simulink model "cm10"  (R2015b)
settings: Solver=VariableStepAuto  StartTime=0.0  StopTime=100  RelTol=1e-3
settings Model: Creator=Zephyr  LastModifiedBy=Zephyr

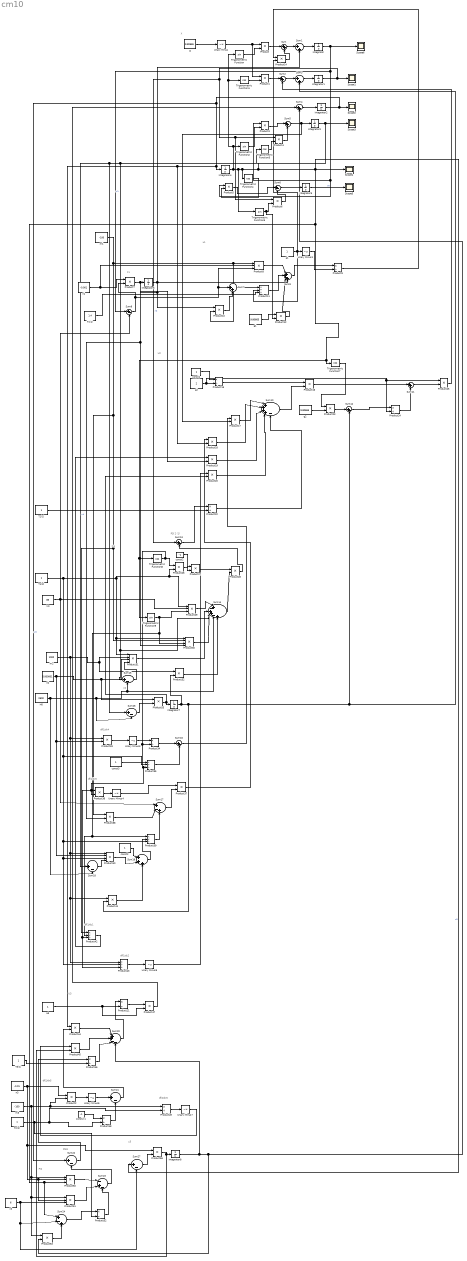
== system cm10 ==
  note: u1
  note: z3
  note: z2
  note: z1
  note: FI2
  note: PSI3
  note: dfi2/dx5
  note: dfi2/dx5
  note: U3
  note: dfi1/dz2
  note: dfi1/dz1
  note: dfi1/dx5
  note: dfi1/dx4
  note: FI1
  note: PSI 2 (1)
  note: U2
  note: X
  H0 : Constant  Value=2600
  Integrator{,1..8} (9 alike) : Integrator
  Product{,1..7,10,12,14,16..20,23,25..28,32..33,36..38,41,44..45,47,53,55..56} (33 alike) : Product
  Product11 : Product  Inputs=*//
  Product{9,15,21..22,24,34,46,48..49,52} (10 alike) : Product  Inputs=*/
  Product{8,29,50..51} (4 alike) : Product  Inputs=3
  Product30 : Product  Inputs=4
  Product31 : Product  Inputs=4
  Product35 : Product  Inputs=*//
  Product39 : Product  Inputs=**/
  Product40 : Product  Inputs=4
  Product42 : Product  Inputs=**/
  Product43 : Product  Inputs=*//
  Scope{1..6} (6 alike) : Scope
  Sum{,1..5,7,11} (8 alike) : Sum  Inputs=|++
  Sum10 : Sum  Inputs=|++++-
  Sum{6,8,12..13,15..16,18,21..22,26..27} (11 alike) : Sum  Inputs=|+-
  Sum14 : Sum  Inputs=|+-++-+
  Sum17 : Sum  Inputs=|+-+
  Sum19 : Sum  Inputs=|+++
  Sum20 : Sum  Inputs=|++--
  Sum23 : Sum  Inputs=|-+-
  Sum24 : Sum  Inputs=|+-+
  Sum9 : Sum  Inputs=|++-+
  T1(1) : Constant  Value=1.4
  T1(2) : Constant
  T2(1) : Constant
  T2(2) : Constant
  T3(1) : Constant
  Trigonometric Function{,2,5,9} (4 alike) : Trigonometry
  Trigonometric Function{1,3..4,7..8} (5 alike) : Trigonometry  Operator=cos
  Unary Minus{,1,3..7} (7 alike) : UnaryMinus
  V0 : Constant  Value=85
  a1 : Constant
  a2 : Constant  Value=2
  a3 : Constant
  const1 : Constant
  const2 : Constant
  "const2 " : Constant  Value=-1
  const2 1 : Constant  Value=-1
  const3 : Constant
  g : Constant  Value=9.80665
  g1 : Constant  Value=9.80665
  g2 : Constant  Value=9.80665
  m1 : Constant  Value=-100
  m2 : Constant  Value=1000
  m3 : Constant  Value=-100
  n1 : Constant  Value=-0.001
  n2 : Constant  Value=0.000001
  n3 : Constant  Value=-0.01
  v0 : Constant  Value=6
  wires:
  g/1 -> Unary Minus/1
  Unary Minus/1 -> Product1/1, Product/1
  Trigonometric Function/1 -> Product/2
  Product/1 -> Sum/1
  Sum/1 -> Sum1/1
  Integrator/1 -> Scope6/1, Sum8/1, Product5/1, Product3/1  "x1"
  Trigonometric Function1/1 -> Product1/2
  Product1/1 -> Sum2/1
  Sum2/1 -> Sum3/1
  Sum3/1 -> Integrator1/1
  Integrator1/1 -> Sum13/1, Product6/1, Product4/1, Scope1/1  "x2"
  Sum4/1 -> Integrator2/1
  Integrator2/1 -> Sum22/1, Product44/1, Product18/2, Integrator4/1, Scope2/1  "x3"
  Trigonometric Function2/1 -> Product3/2
  Product3/1 -> Sum5/1
  Product4/1 -> Sum5/2
  Trigonometric Function3/1 -> Product4/2
  Sum5/1 -> Product17/2, Integrator3/1
  Integrator3/1 -> Sum26/1, Sum18/1, Sum14/4, Sum15/1, Scope3/1  "x4"
  Integrator4/1 -> Trigonometric Function5/1, Trigonometric Function4/1, Trigonometric Function3/1, Sum24/1, Product50/3, Trigonometric Function7/1, Trigonometric Function9/1, Trigonometric Function8/1, Sum27/1, Scope4/1, Trigonometric Function2/1, Trigonometric Function1/1, Trigonometric Function/1  "x5"
  Trigonometric Function4/1 -> Product5/2
  Product5/1 -> Sum6/1
  Trigonometric Function5/1 -> Product12/2, Product6/2
  Product6/1 -> Sum6/2
  Sum6/1 -> Integrator5/1
  n1/1 -> Product8/2, Product7/1
  Product14/1 -> Sum/2
  a2/1 -> Product25/1, Product24/2, Product15/2
  const1/1 -> Product15/1
  Product15/1 -> Product16/1
  Product17/1 -> Sum10/1
  Product18/1 -> Sum10/2
  Sum10/1 -> Product16/2
  Product19/1 -> Sum10/3
  Product20/1 -> Sum10/4
  T2(1)/1 -> Product22/2
  Product22/1 -> Sum10/5
  Product16/1 -> Sum11/1
  g2/1 -> Product23/2
  Trigonometric Function7/1 -> Product23/1
  Product23/1 -> Sum12/1
  Sum12/1 -> Product24/1
  Product24/1 -> Sum11/2
  Sum11/1 -> Product25/2
  Product25/1 -> Sum2/2
  Sum13/1 -> Product22/1
  Trigonometric Function8/1 -> Product43/3, Product42/3, Product36/2, Product36/1, Product35/3, Product34/2, Product26/1
  Product26/1 -> Product27/2
  "const2 "/1 -> Product27/1
  Product27/1 -> Product28/1
  V0/1 -> Sum8/2, Sum17/1, Product29/2
  Trigonometric Function9/1 -> Product39/1, Product42/2, Product30/3, Product29/3
  Product28/1 -> Sum13/2
  Product29/1 -> Sum14/1
  Product30/1 -> Sum14/2
  m2/1 -> Product43/1, Product41/1, Product40/1, Product33/1, Product32/1, Product31/2
  H0/1 -> Sum18/2, Sum26/2, Sum14/5, Sum15/2
  n2/1 -> Product40/2, Product33/2, Product55/1, Product31/3
  Sum15/1 -> Product31/4
  Product31/1 -> Sum14/3
  Product32/1 -> Sum14/6
  Sum14/1 -> Product28/2
  Product33/1 -> Unary Minus3/1
  Unary Minus3/1 -> Product34/1
  Product34/1 -> Sum16/1
  const3/1 -> Product35/1
  T1(2)/1 -> Product43/2, Product40/3, Product39/3, Product35/2, Product29/1, Product26/2, Product31/1, Product30/1
  Product35/1 -> Sum16/2
  Sum16/1 -> Product17/1
  Product36/1 -> Unary Minus4/1
  Unary Minus4/1 -> Product37/1
  Sum17/1 -> Product37/2
  Product38/1 -> Sum17/2
  Product39/1 -> Sum17/3
  Sum18/1 -> Product40/4
  const2/1 -> Sum19/1
  Product40/1 -> Sum19/2
  Sum19/1 -> Product39/2
  Product41/1 -> Sum19/3
  Product37/1 -> Product18/1
  Product42/1 -> Product19/1
  Product43/1 -> Unary Minus5/1
  Unary Minus5/1 -> Product20/1
  a3/1 -> Product47/2, Product21/2
  Sum20/1 -> Product21/1
  Product44/1 -> Sum20/1
  Product45/1 -> Sum20/2
  Product46/1 -> Sum20/3
  Product21/1 -> Product47/1
  Product47/1 -> Sum4/1
  n3/1 -> Product56/1, Product51/2, Product50/2, Product2/1
  m3/1 -> Product53/1, Product51/1, Product50/1, Product2/2, Product49/1
  Product2/1 -> Unary Minus6/1
  Unary Minus6/1 -> Sum21/1
  Product48/1 -> Sum21/2
  Sum21/1 -> Product44/2
  const2 1/1 -> Product48/1
  T2(2)/1 -> Product52/2, Product49/2, Product48/2
  Product49/1 -> Unary Minus7/1
  Unary Minus7/1 -> Product45/1
  Sum22/1 -> Product46/1
  Product50/1 -> Sum23/1
  Product51/1 -> Sum23/2
  v0/1 -> Sum27/2, Sum24/2, Product51/3
  Sum24/1 -> Product52/1
  Product52/1 -> Sum23/3
  Sum23/1 -> Sum22/2
  Product53/1 -> Sum24/3
  Product7/1 -> Product19/2, Integrator6/1
  Integrator6/1 -> Sum9/4, Product10/1, Product38/2, Product30/4, Sum1/2
  Sum26/1 -> Product55/2
  Product55/1 -> Integrator7/1, Product20/2
  Integrator7/1 -> Product41/2, Sum12/2, Sum3/2, Product32/2
  Sum27/1 -> Product56/2
  Integrator8/1 -> Product53/2, Sum4/2, Sum20/4
  Product56/1 -> Product45/2, Integrator8/1
  T3(1)/1 -> Product46/2
  Product9/1 -> Product14/1
  m1/1 -> Product10/2, Product8/1, Product42/1, Product30/2, Product38/1
  Sum8/1 -> Product8/3, Sum7/1, Product7/2
  Unary Minus1/1 -> Product9/2
  Product10/1 -> Sum7/2
  Sum7/1 -> Product11/1
  a1/1 -> Product14/2, Product11/2, Unary Minus1/1
  T1(1)/1 -> Product11/3
  g1/1 -> Product12/1
  Product8/1 -> Sum9/1
  Product11/1 -> Sum9/2
  Product12/1 -> Sum9/3
  Sum9/1 -> Product9/1
  Integrator5/1 -> Scope5/1  "x6"
  Sum1/1 -> Integrator/1
